simulink model "vibrational_transport_optimal_surface"  (R2023b)
settings: Solver=FixedStepAuto  StartTime=0.0  StopTime=0.3188  FixedStep=0.0001  MaxStep=1e-4  RelTol=1e-7
values from neighbouring files (symbols this model uses):
  F_n = f_n * m_o * 9.81    (= 1.7658)    [experimental_vs_optimal_comparison.m]    (also in parameter_estimation.m = f_n * m_o * g; stick_slip.m = u(6))
  g = 9.81    [experimental_vs_optimal_comparison.m]    (also in parameter_estimation.m)
  m_o = 0.009    [experimental_vs_optimal_comparison.m]    (also in parameter_estimation.m; stick_slip.m = u(5))
  mu_k = 0.59    [experimental_vs_optimal_comparison.m]    (also in parameter_estimation.m = x(1); stick_slip.m = u(8))
  mu_s = 0.72    [experimental_vs_optimal_comparison.m]    (also in parameter_estimation.m; stick_slip.m = u(7))
  v_min = 1e-5    (= 1e-05)    [experimental_vs_optimal_comparison.m]    (also in parameter_estimation.m; stick_slip.m = u(9))
  v_o_init = surface_starting_velocity_double    [experimental_vs_optimal_comparison.m]    (also in parameter_estimation.m = part_vz_init)
  z_o_init = part_z_init    [experimental_vs_optimal_comparison.m]    (also in parameter_estimation.m)
undefined symbols (not defined in the file or in its folder): stick_slip
settings Model: Creator=connor  LastModifiedBy=connor
settings SolverCC: ZeroCrossControl=DisableAll
settings DebuggingCC: InheritedTsInSrcMsg=none

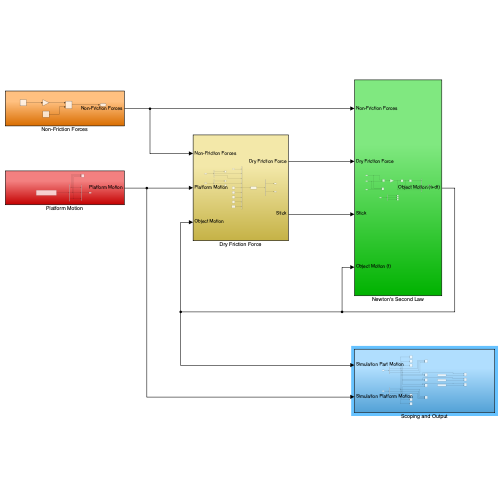
[thumbnail: Simulink's stored preview of the top-level diagram]
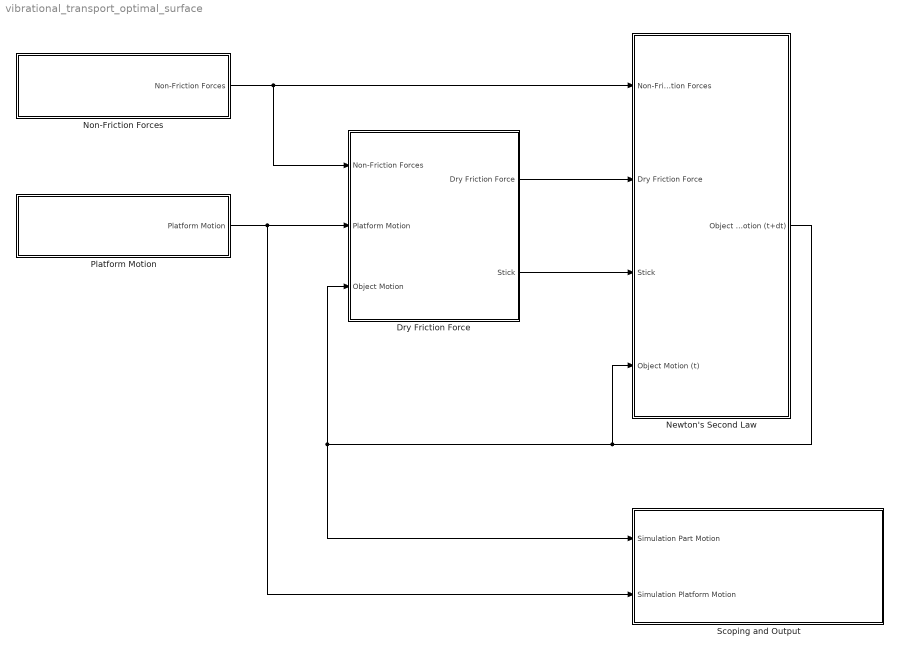
== system vibrational_transport_optimal_surface ==
  Dry Friction Force : Subsystem
  Newton's Second Law : Subsystem
  Non-Friction Forces : Subsystem
  Platform Motion : Subsystem
  Scoping and Output : Subsystem
  wires:
  Platform Motion/1(Platform Motion) -> Scoping and Output/2(Simulation Platform Motion), Dry Friction Force/2(Platform Motion)
  Non-Friction Forces/1(Non-Friction Forces) -> Dry Friction Force/1(Non-Friction Forces), Newton's Second Law/1(Non-Friction Forces)
  Dry Friction Force/1(Dry Friction Force) -> Newton's Second Law/2(Dry Friction Force)
  Dry Friction Force/2(Stick) -> Newton's Second Law/3(Stick)
  Newton's Second Law/1(Object Motion (t+dt)) -> Newton's Second Law/4(Object Motion (t)), Scoping and Output/1(Simulation Part Motion), Dry Friction Force/3(Object Motion)

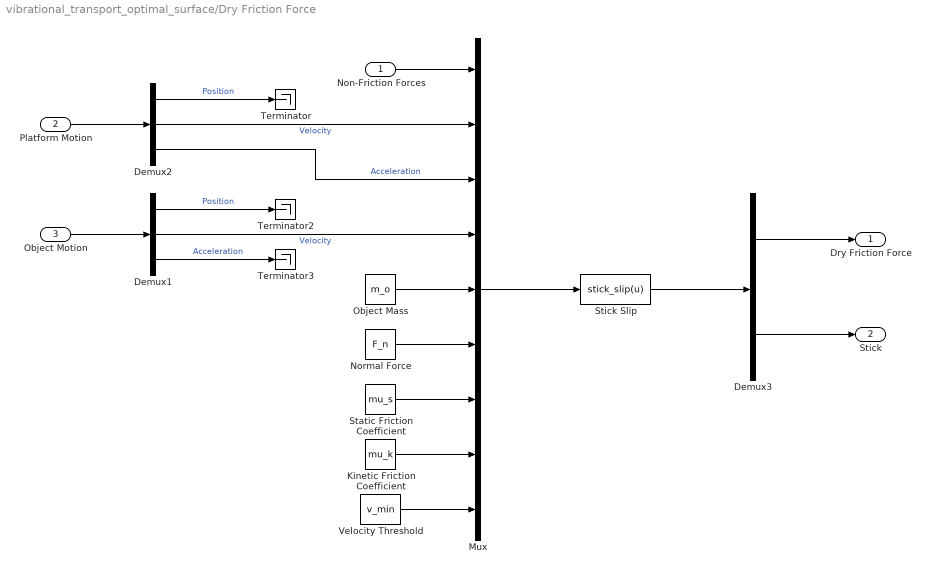
== system vibrational_transport_optimal_surface/Dry Friction Force ==
  Non-Friction Forces : Inport
  Platform Motion : Inport  Port=2
  Object Motion : Inport  Port=3
  Demux1 : Demux  Outputs=3
  Demux2 : Demux  Outputs=3
  Demux3 : Demux  Outputs=2
  Kinetic Friction Coefficient : Constant  Value=mu_k
  Mux : Mux  Inputs=9
  Normal Force : Constant  Value=F_n
  Object Mass : Constant  Value=m_o
  Static Friction Coefficient : Constant  Value=mu_s
  Stick Slip : MATLABFcn  MATLABFcn=stick_slip(u)  OutputDimensions=2
  Terminator : Terminator
  Terminator2 : Terminator
  Terminator3 : Terminator
  Velocity Threshold : Constant  Value=v_min
  Dry Friction Force : Outport
  Stick : Outport  Port=2
  wires:
  Object Motion/1 -> Demux1/1
  Stick Slip/1 -> Demux3/1
  Platform Motion/1 -> Demux2/1
  Mux/1 -> Stick Slip/1
  Demux2/1 -> Terminator/1  "Position"
  Demux2/3 -> Mux/3  "Acceleration"
  Demux2/2 -> Mux/2  "Velocity"
  Demux1/3 -> Terminator3/1  "Acceleration"
  Demux1/2 -> Mux/4  "Velocity"
  Demux1/1 -> Terminator2/1  "Position"
  Velocity Threshold/1 -> Mux/9
  Kinetic Friction Coefficient/1 -> Mux/8
  Object Mass/1 -> Mux/5
  Normal Force/1 -> Mux/6
  Static Friction Coefficient/1 -> Mux/7
  Non-Friction Forces/1 -> Mux/1
  Demux3/1 -> Dry Friction Force/1
  Demux3/2 -> Stick/1

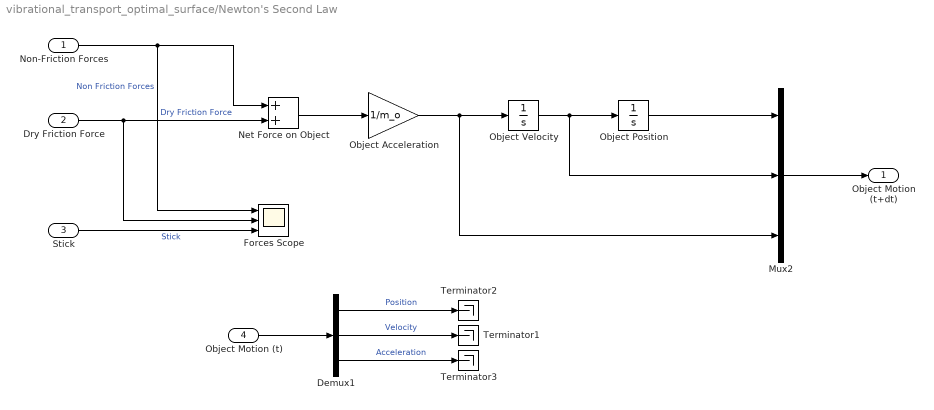
== system vibrational_transport_optimal_surface/Newton's Second Law ==
  Non-Friction Forces : Inport
  Dry Friction Force : Inport  Port=2
  Stick : Inport  Port=3
  Object Motion (t) : Inport  Port=4
  Demux1 : Demux  Outputs=3
  Forces Scope : Scope  NumInputPorts=3
  Mux2 : Mux  Inputs=3
  Net Force on Object : Sum
  Object Acceleration : Gain  Gain=1/m_o
  Object Position : Integrator  InitialCondition=z_o_init
  Object Velocity : Integrator  InitialCondition=v_o_init
  Terminator1 : Terminator
  Terminator2 : Terminator
  Terminator3 : Terminator
  Object Motion (t+dt) : Outport
  wires:
  Object Velocity/1 -> Mux2/2, Object Position/1
  Stick/1 -> Forces Scope/3  "Stick"
  Object Motion (t)/1 -> Demux1/1
  Demux1/2 -> Terminator1/1  "Velocity"
  Demux1/3 -> Terminator3/1  "Acceleration"
  Demux1/1 -> Terminator2/1  "Position"
  Object Acceleration/1 -> Mux2/3, Object Velocity/1
  Net Force on Object/1 -> Object Acceleration/1
  Dry Friction Force/1 -> Net Force on Object/2, Forces Scope/2  "Dry Friction Force"
  Non-Friction Forces/1 -> Net Force on Object/1, Forces Scope/1  "Non Friction Forces"
  Mux2/1 -> Object Motion (t+dt)/1
  Object Position/1 -> Mux2/1

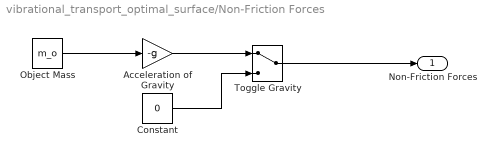
== system vibrational_transport_optimal_surface/Non-Friction Forces ==
  Acceleration of Gravity : Gain  Gain=-g
  Constant : Constant  Value=0
  Object Mass : Constant  Value=m_o
  Toggle Gravity : ManualSwitch
  Non-Friction Forces : Outport
  wires:
  Acceleration of Gravity/1 -> Toggle Gravity/1
  Object Mass/1 -> Acceleration of Gravity/1
  Constant/1 -> Toggle Gravity/2
  Toggle Gravity/1 -> Non-Friction Forces/1

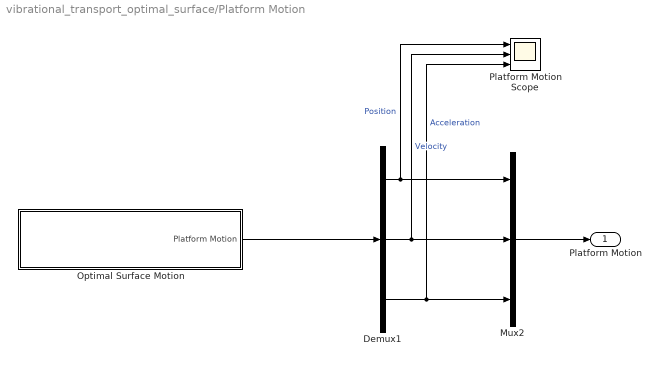
== system vibrational_transport_optimal_surface/Platform Motion ==
  Demux1 : Demux  Outputs=3
  Mux2 : Mux  Inputs=3
  Optimal Surface Motion : Subsystem
  Platform Motion Scope : Scope  NumInputPorts=3
  Platform Motion : Outport
  wires:
  Demux1/3 -> Platform Motion Scope/3, Mux2/3  "Acceleration"
  Demux1/1 -> Platform Motion Scope/1, Mux2/1  "Position"
  Demux1/2 -> Platform Motion Scope/2, Mux2/2  "Velocity"
  Mux2/1 -> Platform Motion/1
  Optimal Surface Motion/1(Platform Motion) -> Demux1/1

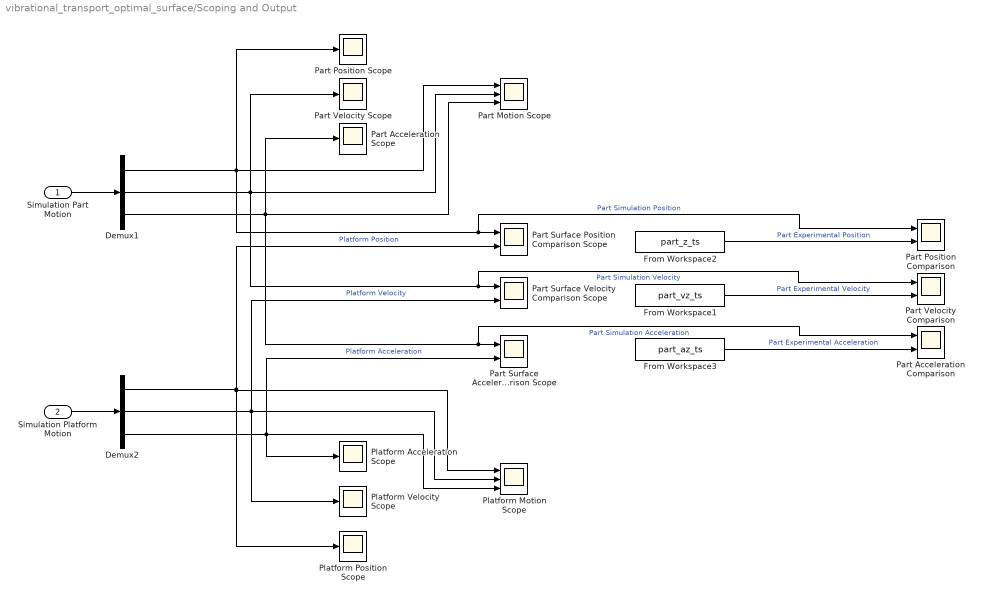
== system vibrational_transport_optimal_surface/Scoping and Output ==
  Simulation Part Motion : Inport
  Simulation Platform Motion : Inport  Port=2
  Demux1 : Demux  Outputs=3
  Demux2 : Demux  Outputs=3
  From Workspace1 : FromWorkspace  VariableName=part_vz_ts  SampleTime=-1
  From Workspace2 : FromWorkspace  VariableName=part_z_ts  SampleTime=-1
  From Workspace3 : FromWorkspace  VariableName=part_az_ts  SampleTime=-1
  Part Acceleration Comparison : Scope  NumInputPorts=2
  Part Acceleration Scope : Scope
  Part Motion Scope : Scope  NumInputPorts=3
  Part Position Comparison : Scope  NumInputPorts=2
  Part Position Scope : Scope
  Part Surface Acceleration Comparison Scope : Scope  NumInputPorts=2
  Part Surface Position Comparison Scope : Scope  NumInputPorts=2
  Part Surface Velocity Comparison Scope : Scope  NumInputPorts=2
  Part Velocity Comparison : Scope  NumInputPorts=2
  Part Velocity Scope : Scope
  Platform Acceleration Scope : Scope
  Platform Motion Scope : Scope  NumInputPorts=3
  Platform Position Scope : Scope
  Platform Velocity Scope : Scope
  wires:
  Simulation Part Motion/1 -> Demux1/1
  Demux1/2 -> Part Velocity Comparison/1, Part Surface Velocity Comparison Scope/1, Part Velocity Scope/1, Part Motion Scope/2  "Part Simulation Velocity"
  Demux1/3 -> Part Acceleration Comparison/1, Part Surface Acceleration Comparison Scope/1, Part Motion Scope/3, Part Acceleration Scope/1  "Part Simulation Acceleration"
  Demux1/1 -> Part Position Comparison/1, Part Surface Position Comparison Scope/1, Part Position Scope/1, Part Motion Scope/1  "Part Simulation Position"
  Simulation Platform Motion/1 -> Demux2/1
  Demux2/2 -> Part Surface Velocity Comparison Scope/2, Platform Motion Scope/2, Platform Velocity Scope/1  "Platform Velocity"
  Demux2/1 -> Platform Motion Scope/1, Platform Position Scope/1, Part Surface Position Comparison Scope/2  "Platform Position"
  Demux2/3 -> Part Surface Acceleration Comparison Scope/2, Platform Motion Scope/3, Platform Acceleration Scope/1  "Platform Acceleration"
  From Workspace2/1 -> Part Position Comparison/2  "Part Experimental Position"
  From Workspace1/1 -> Part Velocity Comparison/2  "Part Experimental Velocity"
  From Workspace3/1 -> Part Acceleration Comparison/2  "Part Experimental Acceleration"

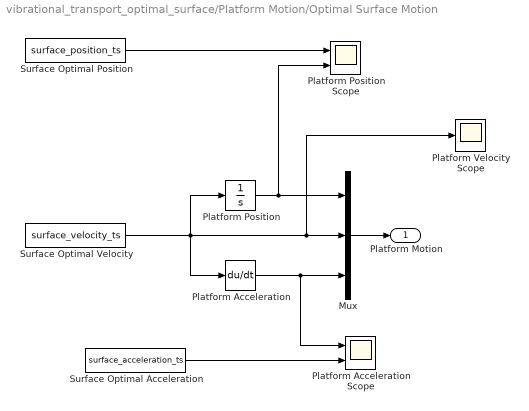
== system vibrational_transport_optimal_surface/Platform Motion/Optimal Surface Motion ==
  Mux : Mux  Inputs=3
  Platform Acceleration : Derivative
  Platform Acceleration Scope : Scope  NumInputPorts=2
  Platform Position : Integrator
  Platform Position Scope : Scope  NumInputPorts=2
  Platform Velocity Scope : Scope
  Surface Optimal Acceleration : FromWorkspace  VariableName=surface_acceleration_ts  SampleTime=-1
  Surface Optimal Position : FromWorkspace  VariableName=surface_position_ts  SampleTime=-1
  Surface Optimal Velocity : FromWorkspace  VariableName=surface_velocity_ts  SampleTime=-1
  Platform Motion : Outport
  wires:
  Platform Acceleration/1 -> Platform Acceleration Scope/1, Mux/3
  Surface Optimal Velocity/1 -> Platform Acceleration/1, Platform Position/1, Platform Velocity Scope/1, Mux/2
  Platform Position/1 -> Platform Position Scope/2, Mux/1
  Surface Optimal Acceleration/1 -> Platform Acceleration Scope/2
  Surface Optimal Position/1 -> Platform Position Scope/1
  Mux/1 -> Platform Motion/1
